simulink library "carnot"  (R2018b)
settings: Solver=VariableStepAuto  StartTime=0.0  StopTime=10.0  RelTol=1e-3
undefined symbols (not defined in the file or in its folder): A, A_earth, acol, Acol, ActPower1, ActPower2, ActPower3, Ad, Ad0, Ar, Au, Au0, Azimuth_Angle, B, Bd, Bd0, Br, Bu, Bu0, C, c1, c2, c3, c33, c4, c5, c6, CarnotCallbacks_Density, CarnotCallbacks_Enthalpy, CarnotCallbacks_Enthalpy2Temperature, CarnotCallbacks_Entropy, CarnotCallbacks_Evaporation_Enthalpy, CarnotCallbacks_GlobalMessageLevel, CarnotCallbacks_Grashof, CarnotCallbacks_Heat_Capacity, CarnotCallbacks_Kinematic_Viscosity, CarnotCallbacks_PMV_PPD, CarnotCallbacks_Prandtl, CarnotCallbacks_Saturation_Property, CarnotCallbacks_Saturation_Temperature, CarnotCallbacks_Saturation_Value_Water, CarnotCallbacks_Specific_Volume, CarnotCallbacks_Thermal_Conductivity, CarnotCallbacks_Vapour_Content, CarnotCallbacks_Vapour_Pressure, Cd, Cdl, Cr, Cu, Davies, Dd, DE_TRY2010_04_averageYear, delta_grd, density, DiameterLastPiece, dl, DPConstant, DPLinear, DPQuadratic, Dr ... (+59)
libraries: $bdroot x429, simulink x36, simulink_extras x12
(part 6 of 22)

== system carnot/Basic/Thermal_Models ==
  Combustion_Calculation : Subsystem  TreatAsAtomicUnit=on
  CreateSdat : Subsystem  mask(CreateSdat){volume=0.5, stgtype=1}
      mask prompts: volume "Volume of storage in m³"; stgtype "Storage Type (0..5)"
      mask help: Create the Sdat structure of the storage (Storage_Type_N). All relevant informations for further evaluation of the storage are combined in this structure. The parameter volume in the storage mask should be promoted from this block.
      mask init:
      | if isempty(volume)||~isnumeric(volume)
      |    volume = 0.1; 
      | end
      | if isempty(stgtype)||~isnumeric(stgtype)
      |    stgtype = 1; 
      | end
      mask Help: web(fullfile(path_carnot('help'),'CreateSdat.html'),'-helpbrowser')
      mask TypeOptions volume: Volume/Value
      mask TypeOptions stgtype: StgType/Value
  Floor_in : Subsystem  mask(inner floor){wallsize=[5 5], t0=20, d=[0.015 0.38 0.02], cond=[1.4 0.79 0.7], cwall=[0.28 0.28 0.28]*3600, rho=[2000 1800 1400], misc=[0.9 0.9], dactive=-1, tau=1000*3600}
      mask prompts: wallsize "size of ceiling [m] [length width]"; t0 "initial temperature [degree centigrade]"; d "thickness of layers [m] (vector) (top to bottom)"; cond "conductivity of layers [W/(m*K)] (vector)"; cwall "capacity of nodes layers  [J/(kg*K)] (vector)"; rho "density of layers [kg/m^3]"; misc "emission_ceiling emission_floor]"; dactive "depth of the active layer(s) in m from upper surface (-1 for none)"; tau "time constant of floor [s]"
      mask help:
      | This is the model of a floor or a ceiling in a house.
      | first element of the vector = top layer (floor for room above)
      | last element of the vector = bottom layer (ceiling for room beneath)
      mask init:
      | h = wallsize(1);
      | w = wallsize(2);
      | wallsurface = h*w;
      | position = [0, 0, 0];
      | nodes = length(d);
      | 
      | emission_c = misc(1);
      | emission_f = misc(2);
      | active = 0;
      | if (dactive>=0) active=1; end
      mask Help: web(fullfile(path_carnot('help'),'Floor_in.html'),'-helpbrowser')
  HeatPump_basic : Subsystem  mask(heat pump){K=[300 -60 1250  -6.67   60   -5.13e-5   306.7   -115 12225], caph=5*4182, capc=5*4182, UA=1}
      mask prompts: K "Parameters K (see also HP_param.m)"; caph "thermal capacity hot loop [J/K]"; capc "thermal capacity cold loop [J/K]"; UA "heat loss coefficient [W/K]"
      mask help:
      | Linearized heat pump model, uses measured data according to EN 14511 as input (Schwamberger, K.: Fortschrittsberichete VDI, Nr. 263, 1991).
      | heating power: Qdot_h = K1*Tcold_in + K2*Thot_out + K3
      | electric power: Pel = K4*Tcold_in + K5*Thot_out + K6
      | source power: Qdot_c = -K7*Tcold_in - K8*Thot_out - K9
      | differential equation: cap*dTh/dt = Qdot + mdot*cp*(T_in-T) + UA*(Tamb-T)
      | with: cap = mass * heat_capactiy
      | See hp_param.m for the parameters K1 to K9.
      mask Help: web(fullfile(path_carnot('help'),'HeatPump_basic.html'),'-helpbrowser')
      mask DialogControl ParameterTabVar0 Prompt: HP Caracteristic
      mask DialogControl ParameterTabVar01 Prompt: Thermal
      mask Display: plot(0,-30,120,130,[30,46,36,46,36,46,30],[40,40,50,60,70,80,80],[70,54,64,54,64,54,64,54,64,54,70],[40,40,44,50,55,60,65,70,75,80,80],[56,45],[95,95],[51,51],[82,95])
  House_OneNodeModel : Subsystem  mask(House One Node Model){A=140, UAout=0.197*(54.6+26.4)+0.286*((45.7+56.0)*2 -(12+4+3+4)), UAin=[1.5 1.5], capa=0.5e6, tini=20, dtroom=inf, AziWin=[0 90 -180 -90], Awin=[12 4 3 4], Uwin=[1    1   1    1]*1.5, Gwin=[1    1   1    1]*0.622*(1-0.15)}
      mask prompts: A "A: heated surface of the house in m²"; UAout "UA: heat loss of walls and roof in W/K"; UAin "UAin: heat transfer to neighbour in W/K"; capa "Cap: thermal capactiy per surface in J/m²/K"; tini "Initial temperature in °C"; dtroom "Max. change of room temperature in K (standard value is 'inf')"; AziWin "Orientation of the 4 windows (south 0, east -90,west 90)"; Awin "Surface of the 4 windows in m² (vector)"; Uwin "Heat loss coefficient of the 4 windows in W/m²/K [vector]"; Gwin "Light transmittance of the 4 windows (0..1) * (1 - frame_part) [vector]"
      mask help:
      | Simple model of 1-node room or house with 4 windows:
      |   (Cap*A) * dT/dt = Qdot_sol + Qdot_int + Qdot_h + UA*(Tamb-T) + UAin*(Tn-T)
      | with
      |   Qdot_sol : Solar gain
      |         = Solar_Radiation * WindowSurface* Light_transmittance * (1-Sunshade)
      |   Sunshade : windows have a shading for solar radiation (no shading = 0) (scalar or vector with 4 elements)
      |   Qdot_int : internal gain in W (typical value is 2.3 W/m² * A)
      |   Qdot_h : power of the heating system in W (positive for heating, negative for cooling
      |   Tamb : ambient outdoor temperature in °C (taken from WDB)
      |   Tn : temperature of neighbour rooms in °C (scalar or vector of length(UAin))
      |
      | Max. change of room temperatue: Set parameter to 0 K to calculate idealized heating behaviour. The power balance (Qdot_all) is the theoretical heating demand (see example_House_Ideal.mdl).
      mask Help: web(fullfile(path_carnot('help'),'HouseOneNodeModel.html'),'-helpbrowser')
      mask TypeOptions A: Troom_calc/A
      mask TypeOptions UAout: UAout/Gain
      mask TypeOptions UAin: UAin/Gain
      mask TypeOptions capa: Troom_calc/capa
      mask TypeOptions tini: Troom_calc/tini
      mask TypeOptions dtroom: Troom_calc/dtroom
      mask TypeOptions Awin: Awin/Value | Awin1/Value
      mask TypeOptions Uwin: Uwin/Value
      mask TypeOptions Gwin: Gwin/Value
      mask DialogControl ParameterTabVar0 Prompt: Geometry
      mask DialogControl ParameterTabVar01 Prompt: Thermal
      mask DialogControl ParameterTabVar012 Prompt: Windows
      mask Display:
      | plot(0,-15,80,100,[30,30,60,60,30],[20,50,50,20,20],...
      |     [47,47,56,56,47],[40,30,30,40,40],...
      |     [42,42,34,34],[20,40,40,20],...
      |     [62,45,28],[48,70,48])
  Pipe_basic : Subsystem  mask(Pipe basic){vol=pi*(0.02/2)^2*10, L=10, uloss=1, effcond=1, cwall=2000, t0=20, nodes=10}
      mask prompts: vol "Volume [m³]"; L "Length of pipe [m]"; uloss "Heat loss per pipe length [W/(m*K)]"; effcond "Effective conductivity of pipe per length [W/(m*K)]"; cwall "Capacity of pipewall per length [J/(m*K)]"; t0 "initial temperature [degree centigrade]"; nodes "number of nodes"
      mask help:
      | Multinode pipe with capacity. The flow is calculated by the upwind scheme heat conduction between nodes by central differences (Patankar 1980).
      | heat loss: u = conductivity / ( d_in * ln (d_out / d_in) )
      mask init:
      | nodes = max(nodes, 1);
      | vnode = max(vol,0.0001)/nodes;
      | lnode = max(L, 0.001)/nodes;
      | cnode = max(0,cwall)*L/vol;
      | unode = uloss*lnode/vnode;
      | cond = effcond/(lnode*lnode);
      mask Help: web(fullfile(path_carnot('help'),'Pipe_basic.html'),'-helpbrowser')
      mask DialogControl ParameterTabVar0 Prompt: Geometry
      mask DialogControl ParameterTabVar01 Prompt: Thermal
      mask DialogControl ParameterTabVar012 Prompt: Calculation
      mask Display: plot(0,0,100,100,[24,27,27,24,75,80,80,75,24,20,20,24],[60,53,46,40,40,46,55,60,60,53,46,40])
  Radiator_basic : Subsystem  mask(basic Radiator){pnomEN=1000, dtnomEN=50, expo=1.3, mcp=4182*1, tini=20}
      mask prompts: pnomEN "Qdot_nom: nominal power in W"; dtnomEN "Tdiff_nom: nominal temperature difference in K"; expo "radiator exponent (> 0)"; mcp "mass * capacity per unit in J/K"; tini "Initial temperature in °C"
      mask help:
      | The block calculates the heat transfer of a radiator to a room according to the EN 442 equation.
      | Qdot = Qdot_nom * (Tdiff/Tdiff_nom)^n
      mask init:
      | mcap = max(1,mcp); % lower limit for capacity is 1 J/K
      | 
      | % correct values because current model 
      | % uses outlet temperature as mean temperature
      | pnom = pnomEN;
      | dtnom = dtnomEN-5;
      mask Help: web(['file:///' fullfile(path_carnot('help'),'Radiator.html')],'-helpbrowser')
  Roof : Subsystem  mask(outer roof){wallsize=[5 5], pos=[0 0 0], t0=20, d=[0.015 0.38 0.02], cond=[1.4 0.79 0.7], cwall=[0.28 0.28 0.28]*3600, rho=[2000 1800 1400], reflectground=0.2, abs_emiss=[0.6, 0.9, 0.9], tau=1000*3600, dactive=-1}
      mask prompts: wallsize "size of wall [m] [height width]"; pos "position [inclination azimuth rotation]"; t0 "initial temperature [degree centigrade]"; d "thickness of nodes [m] (vector)"; cond "conductivity of nodes [W/(m*K)] (vector)"; cwall "capacity of nodes [J/(kg*K)] (vector)"; rho "density [kg/m^3]"; reflectground "reflection of ground"; abs_emiss "[outer absorption, outer emission, inner emisson]"; tau "time-constant of wall [s]"; dactive "depth of active layer in m from outside (-1, if none)"
      mask help:
      | This is the model of an outer roof of a house.
      | first element of the vector = layer to surrounding
      | last element of the vector = layer to room
      mask init:
      | absorption_out = min(1, max(abs_emiss(1),0));
      | nodes = length(d);
      | h = wallsize(1);
      | w = wallsize(2);
      | wallsurface = h*w;
      | emission_c = abs_emiss(3);
      | emission_out = abs_emiss(2);
      | active = 0;
      | if (dactive>=0) active=1; end
      | 
      | %für Variablen in shaderad
      | wallangle = pos(1);
      | wallazimut = pos(2);
      | wallheight=h;
      | wallwidth=w;
      mask Help: web(fullfile(path_carnot('help'),'Roof.html'),'-helpbrowser')
  Room_Node : Subsystem  mask(NODE){zoneairvolume=5*5*2.5, zoneheight=2.5, zonestartTEMP=20, zonestartWATER=55, timeconst=100, heatperfect=natural, lookuptime=[0 24]*3600, lookupvalue=[20 20], AirPressure=101300, calc_p=off}
      mask prompts: zoneairvolume "SIZE: netto air volume >0, m^3"; zoneheight "SIZE: height of zone (floor - ceiling) >0, m"; zonestartTEMP "START TEMPERATURE: convective and radiative node, °C"; zonestartWATER "START AIR HUMIDITY: relative air humidity [0,100], %"; timeconst "timeconstant of radiative and convective node in s"; heatperfect "air temperature"; lookuptime "time vector for ideal profile [s]"; lookupvalue "values for ideal profile [degree centigrade]"; AirPressure "Air pressure for material properties in Pa"; calc_p "Calculate Pressure"
      mask help:
      | This block delivers the energy consumption, temperature and air quality of a zone.
      | It is assumed that this node represents the center of a zone all connected sink and source blocks communicate with. Sink and source blocks are walls, windows, persons, heater etc..
      | Properties of air are calculated once at initialization (with node start temperature, humidity and air pressure).
      | [S] : input vector from sink blocks and source blocks
      | [AIV] : output vector with node temperature and air quality data.
      mask init:
      | CO2norm = 400*1e-6;
      | zoneairvolume = max(0.01, zoneairvolume);
      | zoneheight = max(0.01, zoneheight);
      | zonestartAIR = 10^5*zoneairvolume/(287*(zonestartTEMP+273)); % kg AIR in zone volume
      mask Help: web(fullfile(path_carnot('help'),'Room_Node.html'),'-helpbrowser')
      mask TypeOptions heatperfect: natural | ideal profile (for heating demand)
      mask TypeOptions calc_p: convective_node/Constant1/calc_p
  Solar_Collector_basic : Subsystem  mask(Basic Solar Thermal Collector){acol=acol, c1=c1, c2=c2, c3=c3, c4=c4, c5=c5, c6=c6, tini=tini}
      mask prompts: acol "A : collector surface  [m²]"; c1 "c1 : heat loss coefficient at (Tm-Ta)=0  [W/(m²*K)]"; c2 "c2: temperature dependence of the heat loss coefficient [W/(m*K)²]"; c3 "c3 : wind speed dependence of the heat loss coefficient [J/(m³K)]"; c4 "c4 : sky temperature dependence of the heat loss coefficient [W/(m²K)]"; c5 "c5 : effective thermal capacity [J/(m²K)]"; c6 "c6 : wind dependence in the zero loss efficiency [s/m]"; tini "initial temperature [degree centigrade]"
      mask help: Model according to EN 12975 / ISO 22975
      mask Help: web(fullfile(path_carnot('help'),'Solar_Collector_basic.html'),'-helpbrowser')
      mask Display: disp('solar thermal\ncollector\nEN 12975')
  T_Ground_Undisturbed : Subsystem  mask(Undisturbed ground temperature){Tmeanoutside=0, deltathetae=10, tshift=0, cond_ground=1, rhocp=1000*2000, hh=10, znodes=10}
      mask prompts: Tmeanoutside "mean outside temperature over one year [°C]"; deltathetae "amplitude of monthly outside temperatures [°C]"; tshift "time shift where external temperature sine-curve shows a minimum [h]"; cond_ground "soil thermal conductivity in W/m/K"; rhocp "soil heat capacity per Volume in J/m³/K"; hh "depth z in m"; znodes "number of nodes"
      mask help:
      | The temperature of the undisturbed ground Tg is caclulated for a number of equidistant nodes from the surface down to a depth z.
      |
      | Tg = Tavg - dTavg * exp(-z/dg) * cos(2*pi*(t-ts)/t0 - z/dg) + G*z
      |
      | penetration depth : dg = sqrt(t0*cond/(pi*dens*cp))
      |
      | cond  : thermal conductivity of the ground in W/m/K
      | cp    : heat capacity of the ground in J/kg/K
      | dens  : density of the ground in kg/m³
      | G     : temperature increase in the depth (= 0.03 K/m)
      | t     : time of the year in seconds
      | t0    : total seconds of one year (= 3600*24*365)
      | ts    : time in seconds where the ambient temperature curve shows a minimum
      | Tavg  : annual mean ambient temperature
      | dTavg : annual amplitude of the ambient temperature
      | z     : depth in meters
      |
      | The equation is based on approaches presented in the literature for seasonal temperature variations in the earth’s crust (Baehr & Stephan 2006; Wesselak & Schabbach 2009), neglecting the influence of the heat transfer resistance from the ambient air to the surface of the ground (i.e. u_surf =):
      mask init:
      | %thermische eindringtiefe
      | delta_grd = sqrt((8760*3600*cond_ground)/(pi*rhocp));
      | 
      | % height vector
      | z = [0:hh/znodes:hh];
      mask Help: web(fullfile(path_carnot('help'),'T_Ground_Undisturbed.html'),'-helpbrowser')
      mask Display: plot(0,0,100,100,[90,10],[90,90],[50,50],[-0,90],[49,48,46,44,41,34,25,15],[-0,20,40,50,60,70,80,90],[52,54,56,58,61,67,76,85],[-0,20,40,50,60,70,80,90],[50,49,49,48,48,48,50,54,60],[-0,20,30,40,50,60,70,80,90],[50,51,51,52,52,50,48,43,35],[0,20,30,40,50,60,70,80,90])
  ThermalNodeTHB : Subsystem  mask(Thermal Node){UA=1, mcp=4182, Tini=20}
      mask prompts: UA "UA: thermal loss coefficient in W/K"; mcp "mcp: thermal capacity of the node in J/K"; Tini "Ambient temperature for losses (and initial Temp.) in °C"
      mask help: Thermal node with the THB as input.
      mask Help: web(fullfile(path_carnot('help'),'Thermal_Node.html'),'-helpbrowser')
      mask TypeOptions UA: Thermal_Node/UA
      mask TypeOptions mcp: Thermal_Node/mcp
      mask TypeOptions Tini: Tamb/Value
      mask Display: plot(-20,0,120,100,[10,70,70,10,10],[10,10,70,70,10],[70,90,90,30,10],[10,30,90,90,70],[90,70],[90,70],[50,30],[60,60],[40,40],[30,60])
  Thermal_Node : Subsystem  mask(Thermal Capacity){UA=10, mcp=3*4182}
      mask prompts: UA "UA: thermal loss coefficient in W/K"; mcp "mcp: thermal capacity of the node in J/K"
      mask help:
      | One node model of a thermal mass based on the equation:
      |
      | mcp * dT/dt = UA*(Tamb-T) + mdot*cp_in*(Tin-T) + Qdot
      |
      | cp_in  :  heat capacity of entering fluid in J/kg/K
      | mdot  :  entering fluid massflow in kg/s
      | Qdot  :  additional thermal power added to node in W
      | Tin     :  temperature of entering massflow in °C
      | T        :  temperature of the node in °C
      mask Help: web(fullfile(path_carnot('help'),'Thermal_Node.html'),'-helpbrowser')
      mask TypeOptions UA: Losses/Gain
      mask TypeOptions mcp: nodeCapacity/Value
      mask Display: plot(-20,0,120,100,[10,70,70,10,10],[10,10,70,70,10],[70,90,90,30,10],[10,30,90,90,70],[90,70],[90,70],[50,30],[60,60],[40,40],[30,60])
  Wall_basic : Subsystem  mask(Wall basic){tau=3600, t0=20, d=[0.1 0.1 0.1], dactive=-1, cond=[1 2 1], cwall=[800 1000 800], rho=[2000 2700 2000]}
      mask prompts: tau "Time constant in s"; t0 "Initial temperature in °C"; d "Thickness of layers in m"; dactive "Depth of active layer(s) in m"; cond "Conductivity of layer material in W/m/K"; cwall "Capacity of layer material in J/kg/K"; rho "Density of layer material in kg/m³"
      mask help: Basic model of a wall using a multilayer Beuken model.
      mask Help: web(fullfile(path_carnot('help'),'Wall_basic.html'),'-helpbrowser')
  Wall_in : Subsystem  mask(inner wall){wallsize=[10 10], d=[0.1 0.1 0.1], cond=[1 1 1], cwall=[0.28 0.28 0.28]*3600, rho=[2000 200 2000], emission_in=.96, dactive=[0.075 0.15 0.225], t0=10, tau=10*3600}
      mask prompts: wallsize "size of wall [m] [height width]"; d "thickness of layers [m] (vector) (0 = towards this room)"; cond "conductivity of layers [W/(m*K)] (vector)"; cwall "capacity of layers [J/(kg*K)] (vector)"; rho "density of layers [kg/m³]"; emission_in "emission of wall surface"; dactive "depth active layer in m from inner surface  (-1 = none)"; t0 "initial temperature [degree centigrade]"; tau "time-constant of wall [s]"
      mask help:
      | This is the model of an inner wall in a house.
      | first element of the vector = layer to room ([AIV], [S])
      | last element of the vector = layer to neighbour room ([AIV]n, [S]n)
      mask init:
      | position = [0 90 0 ];
      | % nodes = length(d);
      | wallheight = wallsize(1);
      | wallsurface = wallsize(1)*wallsize(2);
      | 
      | if (dactive>=0) 
      |     active = 1;
      | else
      |     active = 0;
      | end
      mask Help: web(fullfile(path_carnot('help'),'Wall_in.html'),'-helpbrowser')
      mask DialogControl ParameterTabVar0 Prompt: Wall Layers
      mask DialogControl ParameterTabVar01 Prompt: Calculation
  Wall_out : Subsystem  mask(outer wall){wallsize=[2.5 5], pos=180, t0=20, d=[0.1 0.38], cond=[0.04 0.79], cwall=[0.28 0.28]*3600, rho=[900 1800], reflectground=0.2, abs_emiss=[0.65 0.97 0.96], tau=1000*3600, dactive=-1}
      mask prompts: wallsize "size of wall [m] [height width]"; pos "azimut (0=south, east = -90)"; t0 "initial temperature [degree centigrade]"; d "thickness of nodes [m] (vector)"; cond "conductivity of nodes [W/(m*K)] (vector)"; cwall "capacity of nodes [J/(kg*K)] (vector)"; rho "density [kg/m^3]"; reflectground "reflection of ground"; abs_emiss "[outer absorption, outer emission, inner emisson]"; tau "time-constant of wall [s]"; dactive "depth of active layer in m from outside (-1, if none)"
      mask help:
      | This is the model of an outer wall of a house.
      | first element of the vector = layer to surrounding
      | last element of the vector = layer to room
      | The azimut may be a scalar or vector with [inclination azimut rotation], see carnot/Weather/Fixed_Surface.
      mask init:
      | if length(pos) == 1
      |     pos = [90  pos 0]; % pos is [inclination azimut rotation]
      | end
      | absorption_out = min(1, max(abs_emiss(1),0));
      | % nodes = length(d);
      | wallsurface = wallsize(1)* wallsize(2);
      | emission_in = abs_emiss(3);
      | emission_out = abs_emiss(2);
      | active = 0;
      | if (dactive>=0) active=1; end
      | 
      | %für Variablen in shaderad
      | wallangle = pos(1);
      | wallazimut = pos(2);
      | wallheight = wallsize(1);
      | wallwidth = wallsize(2);
      mask Help: web(fullfile(path_carnot('help'),'Wall_out.html'),'-helpbrowser')
  Wall_with_Window : Subsystem  mask(outer wall with window){wallsize=[2.5 5], windowsize=[1 2], frame=0.1, pos=0, t0=20, tau=1000*3600, g=0.7}
      mask prompts: wallsize "size of wall[m] [height width]"; windowsize "size of window[m] [height width]"; frame "part of frame of the window-surface (0..1)"; pos "azimut of wall (0=south, east= -90)]"; t0 "initial temperature [degree centigrade]"; tau "time-constant of wall and window [s]"; g "energy transmission of window"
      mask help:
      | This is the model of an outer wall with window.
      | first element of the vector = layer to surrounding
      | last element of the vector = layer to room
      mask init:
      | pos = [90 pos 0]; % position is [inclination azimut rotation]
      mask Help: web(fullfile(path_carnot('help'),'Wall_with_Window.html'),'-helpbrowser')
  Window : Subsystem  mask(window){pos=0, windowsize=[1 1], frame=0.1, Ug=1.8, gvalue=0.6, tauzero=0.6*0.95, numpanes=2, d=[0.004 0.004], rho=[2500 2500], cp=[1008  1008], t0=20, misc=[0.2 0.1 1 1], shad_type=No shading, type_glazing=double glazing normal, tau_shad=0.01, bli_a=0.05, bli_b=1, bli_c=0.05, bli_d=0.05, bli_alpha=90, bli_refl=0.2}
      mask prompts: pos "azimut (0=south, east = -90)"; windowsize "size of window [m] [height width]"; frame "part of frame of the surface (0..1)"; Ug "heat transfer coefficient (U-value) [W/m²K]"; gvalue "Solar heat gain coefficient (SHGC) [0..1]"; tauzero "Primary solar heat gain (MUST be <= SHGC)"; numpanes "number of glass panes [1..4]"; d "thickness of glass panes [m] (vector with one element per pane)"; rho "density of glass [kg/m³] (vector with one element per pane)"; cp "capacity of glass [J/(kg*K)] (vector with one element per pane)"; t0 "initial temperature [°C]"; misc "[reflection_ground absorption_out emission_out emission_in]"; shad_type "shading type [no Shading/exterior/interior]"; type_glazing "glazing type"; tau_shad "solar transmittance of shading element [0..1]"; bli_a "a  Depth of blind blades [m]"; bli_b "b heigth of blind blades [m]"; bli_c "c distance of "b" to back end of blind blade [m]"; bli_d "d offset between blind blades [m]"; bli_refl "optical reflectance of blind surface [0..1]"
      mask help:
      | The window model evaluates the solar heat gain coefficient and the u-value to build up a two node model. The solar heat gain coefficient (SHGC) is the fraction of solar radiation admitted through a window, door, or skylight -- either transmitted directly and/or absorbed, and subsequently released as heat inside a home. The lower the SHGC, the less solar heat it transmits and the greater its shading ability.  The solar heat gain coefficient (SHGC) consists of two components:
      | + Primary solar heat gain: the solar heat directly transmitted through a glass in its original solar radiation form.
      | + Secondary solar heat gain: the solar heat absorbed by a glass and further transferred to the indoor space as heat by conduction, connection and radiation.
      | Control input [0..1] = fraction of shading (0 - no shading,   1 - full shading)
      mask init:
      | % Geometry
      | h = windowsize(1);
      | w = windowsize(2);
      | windowsurface = h*w;
      | if length(pos) == 1
      |     pos = [90  pos 0]; % pos is [inclination azimut rotation]
      | end
      | 
      | % Optics
      | reflectground = max(0, min(1, misc(1)));
      | absorption_out = max(0, min(1, misc(2)));
      | emission_out = max(0, min(1, misc(3)));
      | emission_in = max(0, min(1, misc(4)));
      | 
      | % Thermal
      | R_norm_in = 1/8;     % h_int = 8 W/m²/K set according to ISO
      | R_norm_out = 1/25;   % h_out = 25 W/m²/K set according to ISO
      | Rwin = 1/Ug - R_norm_in - R_norm_out;
      | % C = sum(cp.*rho.*d.^2); % old equation
      | C = sum(cp.*rho.*d); % corrected equation, hf 29nov2017
      | timeconst = Rwin*C/2;
      mask Help: web(fullfile(path_carnot('help'),'WindowWithShading.html'),'-helpbrowser')
      mask TypeOptions shad_type: alfa_window_in/shad_type
      mask Callback shad_type:
      | switch get_param(gcb,'shad_type')
      |         case 'No shading' % nr. 1 no shading
      |             set_param(gcb,'MaskVisibilities',{'on','on','on','on','on','on','on','on','on','on','on','on','on','off','off','off','off','off','off','off','off'});
      |         case 'Exterior Screen' % nr. 2 external screen
      |             set_param(gcb,'MaskVisibilities',{'on','on','on','on','on','on','on','on','on','on','on','on','on','off','on','off','off','off','off','off','off'});
      |         case 'Interior Screen' % nr. 3 Interior Screen
      |             set_param(gcb,'MaskVisibilities',{'on','on','on','on','on','on','on','on','on','on','on','on','on','on','on','off','off','off','off','off','off'});
      |         case 'Venetian Blind' % nr. 4 venetian blind
      |             set_param(gcb,'MaskVisibilities',{'on','on','on','on','on','on','on','on','on','on','on','on','on','off','off','on','on','on','on','on','on'});
      |     end
      mask TypeOptions type_glazing: alfa_window_in/type_glazing
      mask TypeOptions tau_shad: alfa_window_in/tau_shad
      mask TypeOptions bli_a: alfa_window_in/bli_a
      mask TypeOptions bli_b: alfa_window_in/bli_b
      mask TypeOptions bli_c: alfa_window_in/bli_c
      mask TypeOptions bli_d: alfa_window_in/bli_d
      mask TypeOptions bli_alpha: alfa_window_in/bli_alpha
      mask TypeOptions bli_refl: alfa_window_in/bli_refl
  Window_Optics : Subsystem  mask(Window Optics){BreakpointsForDimension1=[-10 0 50 70 80 90], Table=[1.0 1.0  0.95  0.7  0.0  0.0], Gain=0.8}
      mask prompts: BreakpointsForDimension1 "Breakpoints for the incidence angle in degrees (0° = vertial)"; Table "Energetic transmission of direct sunlight at incidence angle breakpoints [0..1]"; Gain "Energetic light transmission for diffuse sunlight [0..1]"
      mask help: Light transission through the glasses. Data is a combination of glass properties (see taualfa.m) and geometry (shading).
      mask TypeOptions BreakpointsForDimension1: IAM window/BreakpointsForDimension1
      mask TypeOptions Table: IAM window/Table
      mask TypeOptions Gain: IAM diffuse/Gain
  sfunBoiler : S-Function  FunctionName=boiler  Parameters=UA, vol, Tini, nodes  SFunctionDeploymentMode=off  EnableBusSupport=off  mask{UA=0.1, vol=0.01, Tini=20, nodes=1}
      mask prompts: UA "Heat losses in W/K"; vol "Volume (of water) in m³"; Tini "Initial temperature in °C"; nodes "Number of nodes"
      mask init:
      | % set parameters UA,vol,Tini,nodes if empty
      | if isempty(UA)
      |     UA = 1;
      | end
      | if isempty(vol)
      |     vol = 0.01;
      | end
      | if isempty(Tini)
      |     Tini = 20;
      | end
      | if isempty(nodes)
      |     nodes = 20;
      | end
      mask Display:
      | disp('sfunBoiler')
      | port_label('input', 1, 'Tamb')
      | port_label('input', 2, 'Tin')
      | port_label('input', 3, 'mdot')
      | port_label('input', 4, 'p')
      | port_label('input', 5, 'fluid type/mix')
      | port_label('input', 6, 'QdotTherm')
      | port_label('output', 1, 'Tout')
  sfun_storageTnodes : S-Function  FunctionName=storage_Tnodes  Parameters=dia, volume, standing, uloss , ubot, utop, cond, tini, nodes, nconnect, elimthermocline, condinvtc  SFunctionDeploymentMode=off  EnableBusSupport=off  SFcnStateName=DWORK_DH  mask(sfunction storage_Tnodes){uloss=1, ubot=1, utop=1, cond=1, volume=0.5, dia=0.7, standing=standing cylinder, tini=20, nodes=10, nconnect=10, elimthermocline=2, condinvtc=1e5}
      mask prompts: uloss "Heat transfer coefficient to ambient [W/m²K]"; ubot "Heat transfer coefficient to ambient bottom [W/m²K]"; utop "Heat transfer coefficient to ambient top [W/m²K]"; cond "Effective thermal conductivity [W/m/K]"; volume "Volume [m³]"; dia "Diameter [m]"; standing "Position"; tini "Initial temperature in °C"; nodes "Number of nodes"; nconnect "Number of ports"; elimthermocline "Elimination method (0 = off, 1 = temperature dependant, 2 = density dependant)"; condinvtc "COND_ITC: heat transport coefficient for the method 2"
      mask help:
      | The differential equation is derived from the energy conservation equation by using the finite volume method [Patankar: Numerical Heat Transfer and Fluid Flow, 1980].
      | Methods to eliminate the inversed thermocline (It occurs when node with lower density is below a node with higher density. Typically it can be translated to a node with higher temperature below a node with lower temperature. Exception is water below 4°C.):
      | 0 - inversed thermocline is not eliminated
      | 1 - Temperature based: An inversed thermocline exists , if the  temperature of the lower node is more than LIMIT_T_INVERSED degrees  above the upper node. In that case the temperatures of the nodes are mixed. For the geometry of a laying cylinder the different volumes of the nodes are taken in account.
      |  2 - Density based : An inversed thermocline exists, if the density of the lower node is less than the density of the upper node. The model  adds an additional heat transport towards the upper node:
      | heat transport [W/m³] = COND_ITC[W*m³/kg] * density_differnce[kg/m³] / node[m³]
      mask init:
      | if isempty(uloss)
      |     uloss = 1;
      | end
      | 
      | if isempty(ubot)
      |     ubot = 1;
      | end
      | 
      | if isempty(utop)
      |     utop = 1;
      | end
      | 
      | if isempty(cond)
      |     cond = 1;
      | end
      | 
      | if isempty(volume)
      |     volume = 1;
      | end
      | 
      | if isempty(dia)
      |     dia = 1;
      | end
      | 
      | if isempty(standing)
      |     standing = 1;
      | end
      | 
      | if numel(tini) ~= nodes
      |     tini = 20*ones(1,nodes);
      | end
      | 
      | if isempty(nodes)
      |     nodes = 200;
      | end
      | 
      | if isempty(nconnect)
      |     nconnect = 10;
      | end
      | 
      | if isempty(elimthermocline)
      |     elimthermocline = 2;
      | end
      | 
      | if isempty(condinvtc)
      |     condinvtc = 1e5;
      | end
      settings: SFcnIsStateOwnerBlock=on
      mask Help: web(fullfile(path_carnot('help'),'sfun_storageTnodes.html'),'-helpbrowser')
      mask TypeOptions standing: standing cylinder | lying cylinder
      mask DialogControl Container5 Prompt: Thermal
      mask DialogControl Container6 Prompt: Geometry
      mask DialogControl Container7 Prompt: Caclulation
      mask DialogControl Container10 Prompt: Inversed thermocline
      mask Display:
      | disp('storage_Tnodes')
      | 
      | port_label('input', 1, 'Tamb')
      | port_label('output', 1, 'Energy')
      | port_label('output', 2, 'Tnodes')
      | 
      | if exist('nconnect','var')
      |     for n = 1:nconnect
      |         port_label('input',  n+1, ['port' num2str(n)])
      |     end
      | end
  sfun_storage_heatexchanger : Subsystem  mask(storage heat exchanger){idn=finned tube theoretical  - stratified, nodes=10, inlet=10, outlet=1, p1=0, p2=0, p3=0, p4=0, p5=0, p6=0, p7=0}
      mask prompts: idn "type"; nodes "number of nodes"; inlet "inlet node"; outlet "outlet node"; p1 "Parameter 1"; p2 "Parameter 2"; p3 "Parameter 3"; p4 "Parameter 4"; p5 "Parameter 5"; p6 "Parameter 6"; p7 "Parameter 7"
      mask init:
      | switch(idn)
      |     case 1
      |         id = 201;
      |     case 2
      |         id = 301;
      |     case 3
      |         id = 202;
      |     case 4
      |         id = 302;
      |     case 5
      |         id = 203;
      |     case 6
      |         id = 303;
      |     case 7
      |         id = 204;
      |     case 8
      |         id = 304;
      | end
      mask Help: web(['file:///' fullfile(path_carnot('help'),'StoragePorts_HeatExchangerModels.html')],'-helpbrowser')
      mask TypeOptions idn: smooth tube theoretical | smooth tube theoretical - stratified | finned tube theoretical | finned tube theoretical  - stratified | heat transfer from data fit | heat transfer from data fit  - stratified | heat transfer data fit EN12977 | heat transfer data fit EN12977  - stratified

== system carnot/Basic/Weather_and_Sun ==
  Cloudage : Subsystem  mask(cloud index){latitude=51, longitude=-7, longitude0=-30, skytype=high mountain}
      mask prompts: latitude "Latitude [-90;90], north positive"; longitude "Longitude  [-180;180], west positive"; longitude0 "reference longitude (timezone)"; skytype "Sky Type"
      mask help:
      | Calculates the cloud index. The cloud index is the fraction of the sky covered by clouds in [0, 1/8, 2/8, 3/8, ..., 7/8, 1].
      |
      | INPUT VECTOR:
      |  time    : real time or simulation time [s]
      |  Iglob   : global radiation on horizontal surface (W/m²)
      |
      | OUTPUT VECTOR:
      |  cloud  : cloudindex [0;1]
      mask Help: web(fullfile(path_carnot('help'),'Cloudage.html'),'-helpbrowser')
      mask TypeOptions skytype: high mountain | lowland | urban region | industrial zone
  Radiation_Divison : Subsystem  mask(Radiation Division){latitude=52.393800 % Potsdam / Germany, longitude=-13.065100 % Potsdam, longitude0=-15  % CET}
      mask prompts: latitude "Latitude [-90;90], north positive"; longitude "Longitude  [-180;180], west positive"; longitude0 "reference longitude (timezone)"
      mask help:
      | Calculates the direct and diffusive radiation on the horizontal surface as parts of the global radiation.
      |
      | INPUT VECTOR:
      |   time      : real time or simulation time  [s]
      |   Iglob     : global radiation on horizontal surface (W/m²)
      |
      | OUTPUT VECTORS:
      |   Idir           : direct radiation (W/m²)
      |   Idfu          : diffusive radiation (W/m²)
      |   SunAngle
      |   Zenith
      |   Azimuth
      mask Help: web(fullfile(path_carnot('help'),'Radiation_Divison.html'),'-helpbrowser')
  Sky_Temperature : Subsystem  mask(Sky Temperature){tskymodel=on}
      mask prompts: tskymodel "Include time correction (cos-term in Berdahl equation)"
      mask help:
      | Calculates the skytemperature. If humidity data is availabe, the model of Berdahl and Martin 1984 for low clouds (1000 m) is used.
      | Without humidity data, the model of Unsworth with corrected parameters of Feist 1994 is chosen.
      | INPUT VECTOR:
      |   tamb : ambient temperature [°C]
      |   hum  : humidity [%]
      |   cloud: index of cloudness [0,1]
      |
      | OUTPUT VECTOR:
      |   tsky : sky temperature [°C]
      |
      | The calculation can also be used in m-files with the skytemperature.m function.
      mask Help: web(fullfile(path_carnot('help'),'Sky_Temperature.html'),'-helpbrowser')
  Solar_Declination_Angle : Subsystem  mask(solar declination angle){}
      mask help:
      | The block calls the function "solar_declination" in the CARNOT Library
      | Carlib where the calculation is effectuated. The function solar_declination
      | may be used in m-files. The carlib function solar_declination is also
      | used by the "solar_declination"-block in CARNOT.
      | The equation was taken from Duffie, Beckmann: Solar Engineering of
      | Thermal Processes, 2006. Orginaly the equation was derived by Spencer
      | (Spencer: Fourier Series Representation of the Position of the Sun,
      |  Search Vol.2(5), page 172 , 1971). The error is below 0.035°.
      mask Help: web(fullfile(path_carnot('help'),'Solar_Declination_Angle.html'),'-helpbrowser')
  Solar_Extraterrestrial_Radiation : Subsystem  mask(solar extraterrestrial radiation){}
      mask help:
      | The block calls the function "extraterrestrial_radiation" in the CARNOT Library
      | Carlib where the calculation is effectuated. The function solar_extraterrestrial
      | may be used in m-files. The carlib function extraterrestrial_radiation is also
      | used by the "solar_extraterrestrial_radiation"-block in CARNOT.
      | The equation was taken from Duffie, Beckmann: Solar Engineering of
      | Thermal Processes, 2006. Orginaly the equation was derived by Spencer
      | (Spencer: Fourier Series Representation of the Position of the Sun,
      |  Search Vol.2(5), page 172 , 1971). The accuracy is +- 0.01 %
      mask Help: web(fullfile(path_carnot('help'),'Solar_Extraterrestrial_Radiation.html'),'-helpbrowser')
  Solar_Hour_Angle : Subsystem  mask(Solar Hour Angle){timezone=-15, longitude=-7}
      mask prompts: timezone "longitude of timezone (GMT = 0, east negative) in degree"; longitude "longitude of location (east negative) in degree"
      mask help:
      | The block calls the function "solar_hour_angle" in the CARNOT Library
      | Carlib where the calculation is effectuated.
      | The equation was taken from Duffie, Beckmann: Solar Engineering of
      | Thermal Processes, 2006.
      mask Help: web(fullfile(path_carnot('help'),'Solar_Hour_Angle.html'),'-helpbrowser')
  Solar_Position : Subsystem  mask(Solar Position){lati=45, longi=0, timezone=0}
      mask prompts: lati "Geographical latitude in degree (-90..+90, North postive)"; longi "Geographical longitude in degree (-180..+180, West postive)"; timezone "Longitude of timezone in degree (-180..+180, West postive)"
      mask help:
      | Calculate the solar postion (Duffie, Beckman: Solar Engineering of Thermal Processes, 2008).
      | Output is:
      mask Help: web(fullfile(path_carnot('help'),'Solar_Position.html'),'-helpbrowser')
      mask Display: disp('sunpos')
  Solar_Time : Subsystem  mask(solar time){timezone=-15, longitude=-7}
      mask prompts: timezone "longitude of timezone (GMT = 0, east negative) in degree"; longitude "longitude of location (east negative) in degree"
      mask help:
      | The block calls the function "solar_time" in the CARNOT Library
      | Carlib where the calculation is effectuated. The function solar_time
      | may be used in m-files as "solartime2legaltime" or "legaltime2solartime".
      | The carlib function solar_time is also used by the "solar_time"-block in CARNOT.
      | The equation was taken from Duffie, Beckmann: Solar Engineering of
      | Thermal Processes, 2006. Orginaly the equation was derived by Spencer
      | (Spencer: Fourier Series Representation of the Position of the Sun,
      |  Search Vol.2(5), page 172 , 1971). The accuracy is +- 0.01 %
      mask Help: web(fullfile(path_carnot('help'),'Solar_Time.html'),'-helpbrowser')
  WDB_Creator : Subsystem  mask(Weather Data Bus Creator){}
      mask help: Create the weather data bus with scalar inputs.
      mask Help: web(fullfile(path_carnot('help'),'WDB_Creator.html'),'-helpbrowser')

== system carnot/Control/Controller_Bang_Bang ==
  Thot : Inport
  Tcold : Inport  Port=2
  Constant : Constant  Value=Tmax
  MinMax : MinMax  Function=max  Inputs=2  SaturateOnIntegerOverflow=on  InputSameDT=on
  Product : Product  OutDataTypeStr=double  SaturateOnIntegerOverflow=on
  Relational Operator : RelationalOperator  Operator=<=  RndMeth=Nearest  InputSameDT=on
  Relay : Relay  OnSwitchValue=deltaTon  OffSwitchValue=deltaToff
  Sum : Sum  Inputs=-+  SaturateOnIntegerOverflow=on  InputSameDT=on  OutDataTypeStr=Inherit: Same as first input
  control : Outport
  wires:
  Sum/1 -> Relay/1
  Constant/1 -> Relational Operator/2
  Thot/1 -> Sum/2, MinMax/2
  Tcold/1 -> Sum/1, MinMax/1
  MinMax/1 -> Relational Operator/1
  Relay/1 -> Product/1
  Product/1 -> control/1
  Relational Operator/1 -> Product/2

== system carnot/Control/EnergyMeter ==
  note: Shows the power in W and the energy in J gain or loss
      | in a fluid flow (characterised by THB) between the
      | inlet and the outlet of one component.
  THB_out : Inport
  THB_in : Inport  Port=2
  Integrator : Integrator  UpperSaturationLimit=1  LowerSaturationLimit=0
  PowerMeter : $bdroot/Control/PowerMeter
  energy : Outport
  power : Outport  Port=2
  wires:
  THB_out/1 -> PowerMeter/1
  Integrator/1 -> energy/1
  THB_in/1 -> PowerMeter/2
  PowerMeter/1 -> power/1, Integrator/1

== system carnot/Control/EnergyMeter_HC ==
  note: Shows the power in W and the energy in J gain or loss
      | in a fluid flow (characterised by THV) between the
      | inlet and the outlet of one component.
  THB_out : Inport
  THB_in : Inport  Port=2
  Bus Selector : BusSelector  OutputSignals=Temperature
  Bus Selector1 : BusSelector  OutputSignals=Temperature,MassFlow,Pressure,FluidType,FluidMix
  Heat_Capacity : $bdroot/Basic/Material_Properties/Heat_Capacity  VariantControl=CarlibClassic  INPUTARGUMENTS=state variables (classic)  DEBUGLEVEL=DEBUGLEVEL  MAXTOTALWARNINGS=inf  MAXCONSECUTIVEWARNINGS=inf  WRITETOFILE=0  FILENAME='errors.txt'
  Integrator : Integrator  UpperSaturationLimit=1  LowerSaturationLimit=0
  Integrator1 : Integrator  UpperSaturationLimit=1  LowerSaturationLimit=0
  Product : Product  Inputs=***  SaturateOnIntegerOverflow=on  RndMeth=Zero  InputSameDT=on  OutDataTypeStr=Inherit: Same as first input
  T_ave : Gain  Gain=0.5  SaturateOnIntegerOverflow=on  OutDataTypeStr=Inherit: Same as input  ParamDataTypeStr=Inherit: Same as input
  diff_T : Sum  Inputs=+-  SaturateOnIntegerOverflow=on  InputSameDT=on  OutDataTypeStr=Inherit: Same as first input
  only_negative : Saturate  UpperLimit=0  LowerLimit=-inf
  only_positive : Saturate  UpperLimit=inf  LowerLimit=0
  sum : Sum  SaturateOnIntegerOverflow=on  InputSameDT=on  OutDataTypeStr=Inherit: Same as first input
  heating energy : Outport  InitialOutput=0
  power : Outport  Port=2  InitialOutput=0
  cooling energy : Outport  Port=3  InitialOutput=0
  wires:
  THB_in/1 -> Bus Selector/1
  THB_out/1 -> Bus Selector1/1
  Bus Selector1/1 -> diff_T/1, sum/1  "<Temperature>"
  Bus Selector1/4 -> Heat_Capacity/3  "<FluidType>"
  Bus Selector1/5 -> Heat_Capacity/4  "<FluidMix>"
  Heat_Capacity/1 -> Product/1
  Integrator/1 -> heating energy/1
  Bus Selector1/2 -> Product/2  "<MassFlow>"
  diff_T/1 -> Product/3
  Bus Selector/1 -> diff_T/2, sum/2  "<Temperature>"
  sum/1 -> T_ave/1
  T_ave/1 -> Heat_Capacity/1
  Bus Selector1/3 -> Heat_Capacity/2  "<Pressure>"
  Integrator1/1 -> cooling energy/1
  Product/1 -> power/1, only_negative/1, only_positive/1
  only_negative/1 -> Integrator1/1
  only_positive/1 -> Integrator/1

== system carnot/Control/Massflow_Sensor ==
  THB_in : Inport
  Bus Selector : BusSelector  OutputSignals=MassFlow
  heat capacity : StateSpace  A=-tc  B=tc  D=0  InitialCondition=t0
  THB : Outport
  mdot : Outport  Port=2
  wires:
  THB_in/1 -> THB/1, Bus Selector/1
  Bus Selector/1 -> heat capacity/1  "<MassFlow>"
  heat capacity/1 -> mdot/1

== system carnot/Control/Max_Run_Time ==
  In : Inport
  Compare To Zero : simulink/Logic and Bit Operations/Compare To Zero  relop=>  OutDataTypeStr=uint8
  Constant : Constant  Value=-1
  Integrator : Integrator  ExternalReset=rising  InitialCondition=tmaxrun  LimitOutput=on  LowerSaturationLimit=0
  Product : Product  RndMeth=Zero
  Out : Outport
  wires:
  Constant/1 -> Integrator/1
  Integrator/1 -> Compare To Zero/1
  Compare To Zero/1 -> Product/1
  In/1 -> Product/2, Integrator/2
  Product/1 -> Out/1

== system carnot/Control/Min_Run_Time ==
  In : Inport
  Compare To Zero : simulink/Logic and Bit Operations/Compare To Zero  relop=>  OutDataTypeStr=uint8
  Constant : Constant  Value=-1
  Gain : Gain  Gain=mv
  Integrator : Integrator  ExternalReset=rising  InitialCondition=tminrun  LimitOutput=on  LowerSaturationLimit=0
  MinMax : MinMax  Function=max  Inputs=2
  Out : Outport
  wires:
  MinMax/1 -> Out/1
  In/1 -> MinMax/2, Integrator/2
  Compare To Zero/1 -> Gain/1
  Integrator/1 -> Compare To Zero/1
  Constant/1 -> Integrator/1
  Gain/1 -> MinMax/1

== system carnot/Control/Min_Stop_Time ==
  In : Inport
  Compare To Zero : simulink/Logic and Bit Operations/Compare To Zero  relop=<=  OutDataTypeStr=uint8
  Compare To Zero1 : simulink/Logic and Bit Operations/Compare To Zero  relop=<=  OutDataTypeStr=uint8
  Constant : Constant  Value=-1
  Integrator : Integrator  ExternalReset=falling  InitialConditionSource=external  InitialCondition=tminstop  LimitOutput=on  LowerSaturationLimit=0  ShowStatePort=on
  Product : Product  RndMeth=Zero
  Product1 : Product  RndMeth=Zero
  Step : Step  Time=0.1  After=tminstop  SampleTime=0
  Out : Outport
  wires:
  Step/1 -> Integrator/3
  Compare To Zero1/1 -> Product/1
  Integrator/State -> Compare To Zero1/1
  Product/1 -> Integrator/2
  Product1/1 -> Out/1
  In/1 -> Product1/2, Product/2
  Compare To Zero/1 -> Product1/1
  Integrator/1 -> Compare To Zero/1
  Constant/1 -> Integrator/1

== system carnot/Control/PowerMeter ==
  THB_out : Inport
  THB_in : Inport  Port=2
  Bus Selector : BusSelector  OutputSignals=Temperature
  Bus Selector1 : BusSelector  OutputSignals=Temperature,MassFlow,Pressure,FluidType,FluidMix
  Heat_Capacity : $bdroot/Basic/Material_Properties/Heat_Capacity  VariantControl=CarlibClassic  INPUTARGUMENTS=state variables (classic)  DEBUGLEVEL=DEBUGLEVEL  MAXTOTALWARNINGS=inf  MAXCONSECUTIVEWARNINGS=inf  WRITETOFILE=0  FILENAME='errors.txt'
  Product : Product  Inputs=***  SaturateOnIntegerOverflow=on  InputSameDT=on  OutDataTypeStr=Inherit: Same as first input
  T_ave : Gain  Gain=0.5  SaturateOnIntegerOverflow=on  OutDataTypeStr=Inherit: Same as input  ParamDataTypeStr=Inherit: Same as input
  diff_T : Sum  Inputs=+-  SaturateOnIntegerOverflow=on  InputSameDT=on  OutDataTypeStr=Inherit: Same as first input
  sum : Sum  SaturateOnIntegerOverflow=on  InputSameDT=on  OutDataTypeStr=Inherit: Same as first input
  power : Outport
  wires:
  Bus Selector1/1 -> diff_T/1, sum/1  "<Temperature>"
  Bus Selector1/4 -> Heat_Capacity/3  "<FluidType>"
  Bus Selector1/5 -> Heat_Capacity/4  "<FluidMix>"
  Heat_Capacity/1 -> Product/1
  Product/1 -> power/1
  Bus Selector1/2 -> Product/2  "<MassFlow>"
  diff_T/1 -> Product/3
  THB_in/1 -> Bus Selector/1
  Bus Selector/1 -> diff_T/2, sum/2  "<Temperature>"
  sum/1 -> T_ave/1
  T_ave/1 -> Heat_Capacity/1
  Bus Selector1/3 -> Heat_Capacity/2  "<Pressure>"
  THB_out/1 -> Bus Selector1/1

== system carnot/Control/Shading_Control ==
  WDB : Inport
  Troom : Inport  Port=2
  10 minutes lowpass : TransferFcn  Denominator=[600 1]
  Bus Selector1 : BusSelector  OutputSignals=Solar_Radiation_direct_surface,Solar_Radiation_diffuse_surface,Temperature_Ambient
  Compare To Constant : simulink/Logic and Bit Operations/Compare To Constant  relop=>=  const=10  OutDataTypeStr=uint8
  Data Type Conversion : DataTypeConversion
  Hsyt_Solar : Relay  OnSwitchValue=SolarShadeOn  OffSwitchValue=SolarShadeOff  OutDataTypeStr=uint8
  Hyst_Troom : Relay  OnSwitchValue=TroomShadeOn  OffSwitchValue=TroomShadeOff  OutDataTypeStr=uint8
  Logical Operator : Logic  Inputs=3  AllPortsSameDT=off  OutDataTypeStr=boolean
  Saturation : Saturate  UpperLimit=max_shade  LowerLimit=0
  Sum of Elements : Sum  Inputs=2
  Sunshade : Outport
  wires:
  Bus Selector1/3 -> 10 minutes lowpass/1  "<Temperature_Ambient>"
  Bus Selector1/2 -> Sum of Elements/2  "<Solar_Radiation_diffuse_surface>"
  Saturation/1 -> Sunshade/1
  Data Type Conversion/1 -> Saturation/1
  Logical Operator/1 -> Data Type Conversion/1
  Hyst_Troom/1 -> Logical Operator/1
  WDB/1 -> Bus Selector1/1
  Troom/1 -> Hyst_Troom/1
  Compare To Constant/1 -> Logical Operator/3
  Hsyt_Solar/1 -> Logical Operator/2
  Sum of Elements/1 -> Hsyt_Solar/1
  10 minutes lowpass/1 -> Compare To Constant/1
  Bus Selector1/1 -> Sum of Elements/1  "<Solar_Radiation_direct_surface>"

== system carnot/Control/Solar_Radiation_Sensor ==
  WDB : Inport
  Bus Selector : BusSelector  OutputSignals=Solar_Radiation_direct_surface,Solar_Radiation_diffuse_surface
  Idir+Idfu : Sum  Inputs=2  SaturateOnIntegerOverflow=on  InputSameDT=on  OutDataTypeStr=Inherit: Same as first input
  Iglb : Outport
  wires:
  Bus Selector/1 -> Idir+Idfu/1  "<Solar_Radiation_direct_surface>"
  WDB/1 -> Bus Selector/1
  Idir+Idfu/1 -> Iglb/1
  Bus Selector/2 -> Idir+Idfu/2  "<Solar_Radiation_diffuse_surface>"

== system carnot/Control/Start_Delay ==
  In : Inport
  Compare To Zero : simulink/Logic and Bit Operations/Compare To Zero  relop=<=  OutDataTypeStr=uint8
  Constant : Constant  Value=-1
  Integrator : Integrator  ExternalReset=rising  InitialCondition=tstartdelay  LimitOutput=on  LowerSaturationLimit=0
  Product1 : Product  RndMeth=Zero
  Out : Outport
  wires:
  Constant/1 -> Integrator/1
  Integrator/1 -> Compare To Zero/1
  Compare To Zero/1 -> Product1/1
  In/1 -> Product1/2, Integrator/2
  Product1/1 -> Out/1

== system carnot/Control/T_Sensor ==
  THB_in : Inport
  Bus Selector : BusSelector  OutputSignals=Temperature
  heat capacity : StateSpace  A=-tc  B=tc  D=0  InitialCondition=t0
  THB : Outport
  T : Outport  Port=2
  wires:
  THB_in/1 -> THB/1, Bus Selector/1
  Bus Selector/1 -> heat capacity/1  "<Temperature>"
  heat capacity/1 -> T/1

== system carnot/Control/T_Sensor_Surface ==
  note: sensor_node = max(ceil(position*nodes),1)
  Tnodes : Inport
  Constant : Constant  Value=ones(length(pos),1)
  Gain : Gain  Gain=pos  Multiplication=Matrix(u*K)
  Gain1 : Gain  Gain=1/tdel
  Integrator : Integrator  InitialCondition=t0
  MinMax : MinMax  Function=max  Inputs=2
  Rounding Function : Rounding  Operator=ceil
  Selector : Selector  IndexOptions=Index vector (port)  Indices=[1 3]  OutputSizes=1
  Sum : Sum  Inputs=|+-
  Width : Width
  Tsurf : Outport
  wires:
  MinMax/1 -> Selector/2
  Constant/1 -> MinMax/2
  Rounding Function/1 -> MinMax/1
  Gain/1 -> Rounding Function/1
  Selector/1 -> Sum/1
  Integrator/1 -> Tsurf/1, Sum/2
  Sum/1 -> Gain1/1
  Tnodes/1 -> Selector/1, Width/1
  Width/1 -> Gain/1
  Gain1/1 -> Integrator/1
